simulink model "sf_uavmode_template"  (Simulink 5.0)
settings: Solver=ode45  StartTime=0.0  StopTime=10.0  RelTol=1e-3
settings Model: Creator=dlluch  LastModifiedBy=dlluch  BooleanDataType=off

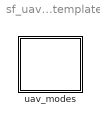
== system sf_uavmode_template ==
  uav_modes : Stateflow chart

== stateflow chart uav_modes ==
  state uav1 [parallel]
    state ac_avoid
      en:mode_count[1][1]++;
    state obs_avoid
      en:mode_count[1][2]++;
    state tgt_aquire
      en:mode_count[1][3]++;
    state form_keep
      en:mode_count[1][4]++;
    uav1 -> ac_avoid : aa
    uav1 -> obs_avoid : oa
    uav1 -> tgt_aquire : ta
    uav1 -> form_keep : fk
    (default) -> ac_avoid
  events: aa local EITHER_EDGE_EVENT; fk local EITHER_EDGE_EVENT; oa local EITHER_EDGE_EVENT; ta local EITHER_EDGE_EVENT
